simulink subsystem "Global_Near_Waypoints"  (R2022b)
settings: Solver=VariableStepAuto  StartTime=0.0  StopTime=10.0  RelTol=1e-3
settings Model: Creator=User  LastModifiedBy=User

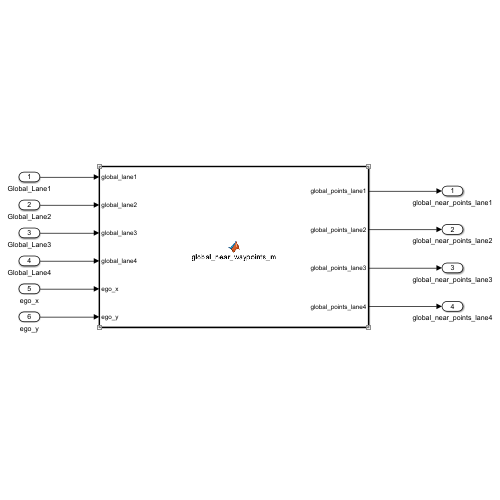
[thumbnail: Simulink's stored preview of the top-level diagram]
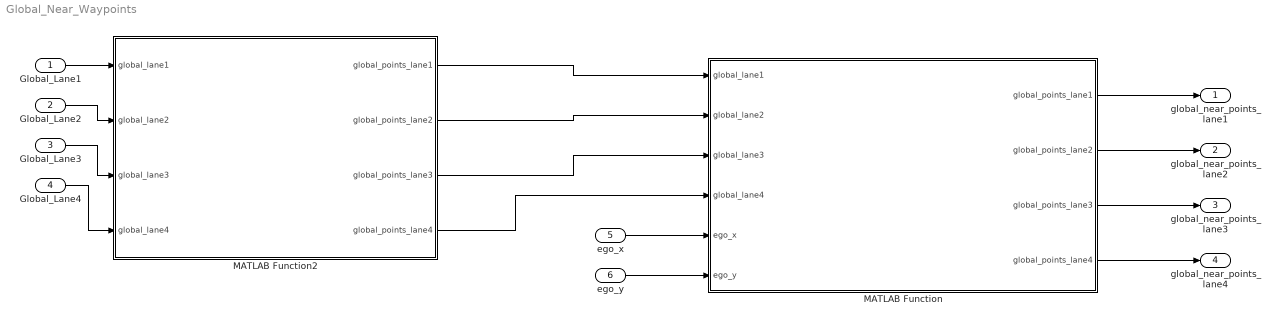
== system Global_Near_Waypoints ==
  Global_Lane1 : Inport
  Global_Lane2 : Inport  Port=2
  Global_Lane3 : Inport  Port=3
  Global_Lane4 : Inport  Port=4
  ego_x : Inport  Port=5
  ego_y : Inport  Port=6
  MATLAB Function : MATLAB Function  TreatAsAtomicUnit=on
  MATLAB Function2 : MATLAB Function  TreatAsAtomicUnit=on
  global_near_points_lane1 : Outport
  global_near_points_lane2 : Outport  Port=2
  global_near_points_lane3 : Outport  Port=3
  global_near_points_lane4 : Outport  Port=4
  wires:
  MATLAB Function/4(global_points_lane4) -> global_near_points_lane4/1
  MATLAB Function/3(global_points_lane3) -> global_near_points_lane3/1
  MATLAB Function/2(global_points_lane2) -> global_near_points_lane2/1
  MATLAB Function/1(global_points_lane1) -> global_near_points_lane1/1
  ego_y/1 -> MATLAB Function/6(ego_y)
  ego_x/1 -> MATLAB Function/5(ego_x)
  Global_Lane1/1 -> MATLAB Function2/1(global_lane1)
  Global_Lane2/1 -> MATLAB Function2/2(global_lane2)
  Global_Lane3/1 -> MATLAB Function2/3(global_lane3)
  Global_Lane4/1 -> MATLAB Function2/4(global_lane4)
  MATLAB Function2/1(global_points_lane1) -> MATLAB Function/1(global_lane1)
  MATLAB Function2/2(global_points_lane2) -> MATLAB Function/2(global_lane2)
  MATLAB Function2/3(global_points_lane3) -> MATLAB Function/3(global_lane3)
  MATLAB Function2/4(global_points_lane4) -> MATLAB Function/4(global_lane4)

== matlab function Global_Near_Waypoints/MATLAB Function ==
  data: global_lane1 input; global_points_lane1 output; global_lane2 input; global_lane3 input; global_lane4 input; ego_x input; ego_y input; global_points_lane2 output; global_points_lane3 output; global_points_lane4 output
function [global_points_lane1, global_points_lane2, global_points_lane3, global_points_lane4] = global_near_waypoints_m(global_lane1, global_lane2, global_lane3, global_lane4, ego_x, ego_y)
    [global_points_lane1, global_points_lane2, global_points_lane3, global_points_lane4] = global_near_waypoints(global_lane1, global_lane2, global_lane3, global_lane4, ego_x, ego_y);
    
end

== matlab function Global_Near_Waypoints/MATLAB Function2 ==
  data: global_lane1 input; global_points_lane1 output; global_points_lane2 output; global_points_lane3 output; global_points_lane4 output; global_lane2 input; global_lane3 input; global_lane4 input
function [global_points_lane1, global_points_lane2, global_points_lane3, global_points_lane4] = get_lane(global_lane1, global_lane2, global_lane3, global_lane4)


persistent lane_road1_value lane_road2_value lane_road3_value lane_road4_value;
    
    % lane_road_value가 비어있으면 처음으로 값을 대입
    if isempty(lane_road1_value)
        lane_road1_value = global_lane1; % 예시: 글로벌 차선 초기 값 line 입력
        lane_road2_value = global_lane2;
        lane_road3_value = global_lane3;
        lane_road4_value = global_lane4;
    end
    % 이후에는 고정된 값을 반환
    global_points_lane1 = lane_road1_value;
    global_points_lane2 = lane_road2_value;
    global_points_lane3 = lane_road3_value;
    global_points_lane4 = lane_road4_value;
end
